simulink model "test_bench"  (R2020a)
settings: Solver=FixedStepDiscrete  StartTime=0.0  StopTime=30.0  FixedStep=Ts  RelTol=1e-3
values from neighbouring files (symbols this model uses):
  Ts = 100e-3    (= 0.1)    [Comparacion.m]    (also in RunTestBench.m; RunTrajectoryControl2.m; RunTrajectoryControlNet.m)
settings Model: Creator=pizarro  LastModifiedBy=charlie
settings DataIOCC: ReturnWorkspaceOutputs=off
settings SFSimCC: CustomCodeUndefinedFunction=UseInterfaceOnly

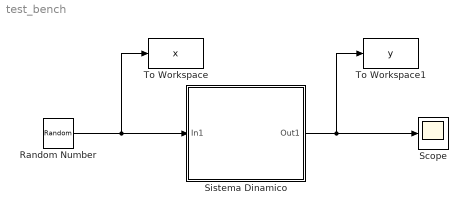
== system test_bench ==
  Random Number : RandomNumber  SampleTime=Ts
  Scope : Scope
  Sistema Dinamico : Subsystem
  To Workspace : ToWorkspace  VariableName=x  SaveFormat=Structure With Time  SampleTime=-1
  To Workspace1 : ToWorkspace  VariableName=y  SaveFormat=Structure With Time  SampleTime=-1
  wires:
  Random Number/1 -> To Workspace/1, Sistema Dinamico/1(In1)
  Sistema Dinamico/1(Out1) -> To Workspace1/1, Scope/1

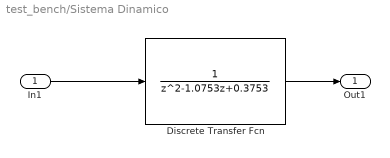
== system test_bench/Sistema Dinamico ==
  In1 : Inport
  Discrete Transfer Fcn : DiscreteTransferFcn  Denominator="[1.0000   -1.0753    0.3753]"  SampleTime=Ts
  Out1 : Outport  VectorParamsAs1DForOutWhenUnconnected=off
  wires:
  Discrete Transfer Fcn/1 -> Out1/1
  In1/1 -> Discrete Transfer Fcn/1
